simulink model "X1PFjicheng"  (R2024a)
settings: Solver=ode3  StartTime=0.0  StopTime=inf  FixedStep=0.05  RelTol=1e-3
undefined symbols (not defined in the file or in its folder): A0, Delta, down, Kdelta, P0, Td, Tj, ud, up, Waypoints, WPNum
libraries: slpidlib x2
(part 2 of 2)

== matlab function X1PFjicheng/AUV动力学模型1/MATLAB Function1 ==
  data: Xjiang input; Xshui input; Yshui input; Zshui input; Kshui input; Mshui input; Nshui input; Xduo input; Yduo input; Zduo input; Kduo input; Mduo input; Nduo input; Xjing input; Yjing input; dot_u output; dot_v output; dot_w output; dot_p output; Zjing input; Kjing input; Mjing input; u input; v input; w input; p input; q input; r input; dot_q output; dot_r output; mass input; Ix input; Iy input; Iz input; Xdot_u input; Ydot_v input; Ydot_p input; Ydot_r input; Zdot_w input; Zdot_q input; Kdot_p input; Kdot_v input; Kdot_r input; Mdot_q input; Mdot_w input; Ndot_v input; Ndot_p input; Ndot_r input
function [dot_u,dot_v,dot_w,dot_p,dot_q,dot_r]= fcn(Xjiang,Xshui,Yshui,Zshui,Kshui,Mshui,Nshui,Xduo,Yduo,Zduo,Kduo,Mduo,Nduo,Xjing,Yjing,Zjing,Kjing,Mjing,u,v,w,p,q,r,mass,Ix,Iy,Iz,Xdot_u,Ydot_v,Ydot_p,Ydot_r,Zdot_w,Zdot_q, ...
    Kdot_p,Kdot_v,Kdot_r,Mdot_q,Mdot_w,Ndot_v,Ndot_p,Ndot_r)

    
    dot_u=-(Xduo + Xjing + Xshui+Xjiang - mass*q*w + mass*r*v)/(Xdot_u - mass);

    dot_v= -(Ix*Iz*Yduo + Ix*Iz*Yjing + Ix*Iz*Yshui - Iz*Kdot_p*Yduo + Iz*Kduo*Ydot_p - Iz*Kdot_p*Yjing + Iz*Kjing*Ydot_p - Iz*Kdot_p*Yshui + Iz*Kshui*Ydot_p - ...
       Ix*Ndot_r*Yduo + Ix*Nduo*Ydot_r - Ix*Ndot_r*Yjing - Ix*Ndot_r*Yshui + Ix*Nshui*Ydot_r + Kdot_p*Ndot_r*Yduo - Kdot_p*Nduo*Ydot_r - Kdot_r*Ndot_p*Yduo + ...
       Kdot_r*Nduo*Ydot_p + Kduo*Ndot_p*Ydot_r - Kduo*Ndot_r*Ydot_p + Kdot_p*Ndot_r*Yjing - Kdot_r*Ndot_p*Yjing + Kjing*Ndot_p*Ydot_r - Kjing*Ndot_r*Ydot_p + ...
       Kdot_p*Ndot_r*Yshui - Kdot_p*Nshui*Ydot_r - Kdot_r*Ndot_p*Yshui + Kdot_r*Nshui*Ydot_p + Kshui*Ndot_p*Ydot_r - Kshui*Ndot_r*Ydot_p + Ix^2*Ydot_r*p*q - Iz^2*Ydot_p*q*r - ...
       Ix*Iy*Ydot_r*p*q - Ix*Kdot_p*Ydot_r*p*q + Ix*Kdot_r*Ydot_p*p*q + Iy*Kdot_p*Ydot_r*p*q - Iy*Kdot_r*Ydot_p*p*q + Iy*Iz*Ydot_p*q*r + Iy*Ndot_p*Ydot_r*q*r - Iy*Ndot_r*Ydot_p*q*r - ...
       Iz*Ndot_p*Ydot_r*q*r + Iz*Ndot_r*Ydot_p*q*r + Ix*Iz*mass*p*w - Ix*Iz*mass*r*u - Iz*Kdot_p*mass*p*w + Iz*Kdot_p*mass*r*u - Ix*Ndot_r*mass*p*w + Ix*Ndot_r*mass*r*u + ...
       Kdot_p*Ndot_r*mass*p*w - Kdot_p*Ndot_r*mass*r*u - Kdot_r*Ndot_p*mass*p*w + Kdot_r*Ndot_p*mass*r*u)/(Ix*Iz*Ydot_v - Iz*Kdot_p*Ydot_v + Iz*Kdot_v*Ydot_p - Ix*Ndot_r*Ydot_v + ...
       Ix*Ndot_v*Ydot_r + Kdot_p*Ndot_r*Ydot_v - Kdot_p*Ndot_v*Ydot_r - Kdot_r*Ndot_p*Ydot_v + Kdot_r*Ndot_v*Ydot_p + Kdot_v*Ndot_p*Ydot_r - Kdot_v*Ndot_r*Ydot_p - Ix*Iz*mass + Iz*Kdot_p*mass + ...
       Ix*Ndot_r*mass - Kdot_p*Ndot_r*mass + Kdot_r*Ndot_p*mass);

    dot_w= -(Iy*Zduo + Iy*Zjing + Iy*Zshui - Mdot_q*Zduo + Mduo*Zdot_q - Mdot_q*Zjing + Mjing*Zdot_q - Mdot_q*Zshui + Mshui*Zdot_q + Mdot_q*mass*p*v - Mdot_q*mass*q*u - Ix*Zdot_q*p*r + ...
       Iz*Zdot_q*p*r - Iy*mass*p*v + Iy*mass*q*u)/(Iy*Zdot_w - Mdot_q*Zdot_w + Mdot_w*Zdot_q - Iy*mass + Mdot_q*mass);
 
    dot_p=-(Iz*Kdot_v*Yduo - Iz*Kduo*Ydot_v + Iz*Kdot_v*Yjing - Iz*Kjing*Ydot_v + Iz*Kdot_v*Yshui - Iz*Kshui*Ydot_v + Kdot_r*Ndot_v*Yduo - Kdot_r*Nduo*Ydot_v - Kdot_v*Ndot_r*Yduo + ...
        Kdot_v*Nduo*Ydot_r + Kduo*Ndot_r*Ydot_v - Kduo*Ndot_v*Ydot_r + Kdot_r*Ndot_v*Yjing - Kdot_v*Ndot_r*Yjing + Kjing*Ndot_r*Ydot_v - Kjing*Ndot_v*Ydot_r + Kdot_r*Ndot_v*Yshui - ...
        Kdot_r*Nshui*Ydot_v - Kdot_v*Ndot_r*Yshui + Kdot_v*Nshui*Ydot_r + Kshui*Ndot_r*Ydot_v - Kshui*Ndot_v*Ydot_r + Iz*Kduo*mass + Iz*Kjing*mass + Iz*Kshui*mass + Kdot_r*Nduo*mass - ...
        Kduo*Ndot_r*mass - Kjing*Ndot_r*mass + Kdot_r*Nshui*mass - Kshui*Ndot_r*mass + Iz^2*Ydot_v*q*r - Iz^2*mass*q*r - Ix*Kdot_r*Ydot_v*p*q + Ix*Kdot_v*Ydot_r*p*q + Iy*Kdot_r*Ydot_v*p*q - ...
        Iy*Kdot_v*Ydot_r*p*q - Iy*Iz*Ydot_v*q*r + Iy*Ndot_r*Ydot_v*q*r - Iy*Ndot_v*Ydot_r*q*r - Iz*Ndot_r*Ydot_v*q*r + Iz*Ndot_v*Ydot_r*q*r + Ix*Kdot_r*mass*p*q - Iy*Kdot_r*mass*p*q + ...
        Iy*Iz*mass*q*r - Iy*Ndot_r*mass*q*r + Iz*Ndot_r*mass*q*r + Iz*Kdot_v*mass*p*w - Iz*Kdot_v*mass*r*u + Kdot_r*Ndot_v*mass*p*w - Kdot_r*Ndot_v*mass*r*u - Kdot_v*Ndot_r*mass*p*w + ...
        Kdot_v*Ndot_r*mass*r*u)/(Ix*Iz*Ydot_v - Iz*Kdot_p*Ydot_v + Iz*Kdot_v*Ydot_p - Ix*Ndot_r*Ydot_v + Ix*Ndot_v*Ydot_r + Kdot_p*Ndot_r*Ydot_v - Kdot_p*Ndot_v*Ydot_r - Kdot_r*Ndot_p*Ydot_v + ...
        Kdot_r*Ndot_v*Ydot_p + Kdot_v*Ndot_p*Ydot_r - Kdot_v*Ndot_r*Ydot_p - Ix*Iz*mass + Iz*Kdot_p*mass + Ix*Ndot_r*mass - Kdot_p*Ndot_r*mass + Kdot_r*Ndot_p*mass);
 
    dot_q=-(Mdot_w*Zduo - Mduo*Zdot_w + Mdot_w*Zjing - Mjing*Zdot_w + Mdot_w*Zshui - Mshui*Zdot_w + Mduo*mass + Mjing*mass + Mshui*mass - Mdot_w*mass*p*v + Mdot_w*mass*q*u + Ix*Zdot_w*p*r - ...
        Iz*Zdot_w*p*r - Ix*mass*p*r + Iz*mass*p*r)/(Iy*Zdot_w - Mdot_q*Zdot_w + Mdot_w*Zdot_q - Iy*mass + Mdot_q*mass);

   dot_r= -(Ix*Ndot_v*Yduo - Ix*Nduo*Ydot_v + Ix*Ndot_v*Yjing + Ix*Ndot_v*Yshui - Ix*Nshui*Ydot_v - Kdot_p*Ndot_v*Yduo + Kdot_p*Nduo*Ydot_v + Kdot_v*Ndot_p*Yduo - Kdot_v*Nduo*Ydot_p - ...
       Kduo*Ndot_p*Ydot_v + Kduo*Ndot_v*Ydot_p - Kdot_p*Ndot_v*Yjing + Kdot_v*Ndot_p*Yjing - Kjing*Ndot_p*Ydot_v + Kjing*Ndot_v*Ydot_p - Kdot_p*Ndot_v*Yshui + Kdot_p*Nshui*Ydot_v + Kdot_v*Ndot_p*Yshui - ...
       Kdot_v*Nshui*Ydot_p - Kshui*Ndot_p*Ydot_v + Kshui*Ndot_v*Ydot_p + Ix*Nduo*mass + Ix*Nshui*mass - Kdot_p*Nduo*mass + Kduo*Ndot_p*mass + Kjing*Ndot_p*mass - Kdot_p*Nshui*mass + Kshui*Ndot_p*mass - ...
       Ix^2*Ydot_v*p*q + Ix^2*mass*p*q + Ix*Iy*Ydot_v*p*q + Ix*Kdot_p*Ydot_v*p*q - Ix*Kdot_v*Ydot_p*p*q - Iy*Kdot_p*Ydot_v*p*q + Iy*Kdot_v*Ydot_p*p*q - Iy*Ndot_p*Ydot_v*q*r + Iy*Ndot_v*Ydot_p*q*r + Iz*Ndot_p*Ydot_v*q*r - ...
       Iz*Ndot_v*Ydot_p*q*r - Ix*Iy*mass*p*q - Ix*Kdot_p*mass*p*q + Iy*Kdot_p*mass*p*q + Iy*Ndot_p*mass*q*r - Iz*Ndot_p*mass*q*r + Ix*Ndot_v*mass*p*w - Ix*Ndot_v*mass*r*u - Kdot_p*Ndot_v*mass*p*w + Kdot_p*Ndot_v*mass*r*u + ...
       Kdot_v*Ndot_p*mass*p*w - Kdot_v*Ndot_p*mass*r*u)/(Ix*Iz*Ydot_v - Iz*Kdot_p*Ydot_v + Iz*Kdot_v*Ydot_p - Ix*Ndot_r*Ydot_v + Ix*Ndot_v*Ydot_r + Kdot_p*Ndot_r*Ydot_v - Kdot_p*Ndot_v*Ydot_r - Kdot_r*Ndot_p*Ydot_v + ...
       Kdot_r*Ndot_v*Ydot_p + Kdot_v*Ndot_p*Ydot_r - Kdot_v*Ndot_r*Ydot_p - Ix*Iz*mass + Iz*Kdot_p*mass + Ix*Ndot_r*mass - Kdot_p*Ndot_r*mass + Kdot_r*Ndot_p*mass);
 

	
end

== matlab function X1PFjicheng/AUV运动学模型1/MATLAB Function ==
  data: u input; ksi_dot output; v input; w input; phi input; theta input; psi input; eta_dot output; zeta_dot output
function [ksi_dot,eta_dot, zeta_dot] = fcn(u,v,w,phi,theta,psi)
ksi_dot=u*cos(psi)*cos(theta)+v*(cos(psi)*sin(theta)*sin(phi)-sin(psi)*cos(phi))+w*(sin(theta)*cos(psi)*sin(phi)+sin(psi)*sin(phi));
eta_dot=u*sin(psi)*cos(theta)+v*(sin(psi)*sin(theta)*sin(phi)+cos(phi)*cos(psi))+w*(sin(theta)*sin(psi)*cos(phi)-cos(psi)*sin(phi));
zeta_dot=-u*sin(theta)+v*cos(theta)*sin(phi)+w*cos(theta)*cos(phi);

end

== matlab function X1PFjicheng/Heading Autopilot/MATLAB Function3 ==
  data: in input; u output
function u = OrientationErrorDegSat(in)
if in > 180
    u = in - 360;
elseif in<-180
    u = in+360;
else
    u = in;
end

== matlab function X1PFjicheng/Compass/MATLAB Function ==
  data: in input; u output
function u = OrientationDegSat(in)
if in > 360
    u = in - 360;
elseif in<0
    u = in+360;
else
    u = in;
end

== matlab function X1PFjicheng/AUV动力学模型1/MATLAB Function2 ==
  data: p input; deg_p output; q input; r input; deg_q output; deg_r output
function [deg_p,deg_q,deg_r]= fcn(p,q,r)
deg_p=rad2deg(p);
deg_q=rad2deg(q);
deg_r=rad2deg(r);

== matlab function X1PFjicheng/卡舵设定/MATLAB Function ==
  data: u input; y output
function y = fcn(u)

y = deg2rad(u);

== matlab function X1PFjicheng/AUV动力学模型1/静力 ==
  data: P input; Xjing output; B input; theta input; Yjing output; Zjing output; Kjing output; Mjing output; phi input; Zg input; Zb input
 
function [Xjing,Yjing,Zjing,Kjing,Mjing]= fcn(P,B,theta,phi,Zg,Zb)

Xjing = -(P-B)*sin(theta);
Yjing = (P-B)*cos(theta)*sin(phi);
Zjing = (P-B)*cos(theta)*cos(phi);
Kjing = -(Zg*P-Zb*B)*cos(theta)*sin(phi);
Mjing =-(Zg*P-Zb*B)*sin(theta);

== matlab function X1PFjicheng/AUV动力学模型1/水动力1/MATLAB Function ==
  data: Xqq input; Xrr input; Xrp input; Xvr input; Xwq input; Xuu input; Xvv input; Xww input; Yp_p input; Ypq input; Yqr input; Yvq input; Ywp input; Ywr input; Yr input; Yp input; Yv_r input; Y0 input; Yv input; Yv_v input; Yvw input; Zpp input; Zrr input; Zrp input; Zvr input; Zvp input; Zq input; Zw_q input; Z0 input; Zw input; Zw_w input; Z_w input; Zww input; Kqr input; Kpq input; Kp_p input; Kp input; Kr input; Kvq input; Kwp input; Kwr input; K0 input; Kv input; Kv_v input; Kvw input; Mpp input; Mrr input; Mrp input; Mq_q input; Mvr input; Mvp input; Mq input; M_wq input; M0 input; Mw input; Mw_w input; M_w input; Mww input; Mvv input; Npq input; Nqr input; Nr_r input; Nwr input; Nwp input; Nvq input; Np input; Nr input; N_vr input; N0 input; Nv input; Nv_v input; Nvw input; u input; Xshui output; v input; w input; p input; q input; r input; Yshui output; Zshui output; Kshui output; Mshui output; Nshui output; rou input; L input
function [Xshui,Yshui,Zshui,Kshui,Mshui,Nshui]= fcn(Xqq,Xrr,Xrp,Xvr,Xwq,Xuu,Xvv,Xww, ...
    Yp_p ,Ypq,Yqr,Yvq,Ywp,Ywr,Yr,Yp,Yv_r ,Y0,Yv,Yv_v ,Yvw, ...
   Zpp,Zrr,Zrp,Zvr,Zvp,Zq,Zw_q,Z0,Zw,Zw_w,Z_w,Zww, ...
    Kqr,Kpq,Kp_p,Kp,Kr,Kvq,Kwp,Kwr,K0,Kv,Kv_v,Kvw, ...
  Mpp,Mrr,Mrp,Mq_q,Mvr,Mvp,Mq,M_wq,M0,Mw,Mw_w,M_w,Mww,Mvv, ...
    Npq,Nqr,Nr_r,Nwr,Nwp,Nvq,Np,Nr,N_vr,N0,Nv,Nv_v,Nvw, ...
    u,v,w,p,q,r,rou,L)
Xshui=0.5*rou*L^4*(Xqq*q ^2+Xrr*r^2+Xrp*r*p)+0.5*rou*L^3*(Xvr*v*r*+Xwq*w*q)+0.5*rou*L^2*(Xuu*u*u+Xvv*v*v+Xww*w*w);
Yshui=0.5*rou*L^4*(Yp_p*p*abs(p)+Ypq*p*q+Yqr*q*r)+0.5*rou*L^3*(Yvq*v*q+Ywp*w*p+Ywr*w*r)+0.5*rou*L^3*(Yr*u*r+Yp*u*p+Yv_r*sign(v)*abs(sqrt(v^2+w^2))*abs(r))+0.5*rou*L^2*(Y0*u*u+Yv*u*v+Yv_v*v*abs(sqrt(v^2+w^2))+Yvw*v*w);
Zshui=0.5*rou*L^4*(Zpp*p*p+Zrr*r*r+Zrp*r*p)+0.5*rou*L^3*(Zvr*v*r+Zvp*v*p)+0.5*rou*L^3*(Zq*u*q+Zw_q*sign(w)*abs(sqrt(v^2+w^2))*abs(q))+0.5*rou*L^2*(Z0*u*u+Zw*u*w+Zw_w*w*abs(sqrt(v^2+w^2)) +Z_w*u*abs(w)+Zww*abs(w*sqrt(v^2+w^2)));
Kshui=0.5*rou*L^5*(Kqr*q*r+Kpq*p*q+Kp_p*p*abs(p))+0.5*rou*L^4*(Kp*u*p+Kr*u*r+Kvq*v*q+Kwp*w*p+Kwr*w*r)+0.5*rou*L^3*(K0*u*u+Kv*u*v+Kv_v*v*abs(sqrt(v^2+w^2))+Kvw*v*w);
Mshui=0.5*rou*L^5*(Mpp*p*p+Mrr*r*r+Mrp*r*p+Mq_q*q*abs(q))+0.5*rou*L^4*(Mvr*v*r+Mvp*v*p+Mq*u*q+M_wq*abs(sqrt(v^2+w^2))*q)+0.5*rou*L^3*(M0*u*u+Mw*u*w+Mw_w*w*abs(sqrt(v^2+w^2))+M_w*u*abs(w)+Mww*abs(w*sqrt(v^2+w^2))+Mvv*v*v);
Nshui=0.5*rou*L^5*(Npq*p*q+Nqr*q*r+Nr_r*r*abs(r))+0.5*rou*L^4*(Nwr*w*r+Nwp*w*p+Nvq*v*q+Np*u*p+Nr*u*r+N_vr*abs(sqrt(v^2+w^2))*r)+0.5*rou*L^3*(N0*u*u+Nv*u*v+Nv_v*v*abs(sqrt(v^2+w^2))+Nvw*v*w);

== matlab function X1PFjicheng/卡舵设定/MATLAB Function4 ==
  data: u input; y output
function y = fcn(u)

y = deg2rad(u);

== matlab function X1PFjicheng/Coupled3DLOS/CoupledLOS ==
  data: ye input; ze input; R_FN input; delta_max input; delta_min input; nanmda input; Gamma_d output; Chi_d output; min input; max input; Delta output
function [Gamma_d,Chi_d,Delta] = fcn(ye,ze,R_FN,delta_max,delta_min,nanmda,min,max)

if ye>min && ye<max
Delta=(delta_max-delta_min)*exp(-nanmda*ye^2)+delta_min;
elseif ye<=min 
    Delta=delta_min;
else 
    Delta=delta_max;
end

LOS_F = [Delta;ye;ze];
LOS_N = R_FN*LOS_F;
Gamma_d = atan2(LOS_N(2),LOS_N(1));
%Gamma_d = atan2(LOS_N(2),sign(LOS_N(1))*sqrt(LOS_N(1)*LOS_N(1)+LOS_N(3)*LOS_N(3)));
if Gamma_d<0
    Gamma_d = Gamma_d+2*pi;
end
Gamma_d = Gamma_d*180/pi;
Chi_d = -atan(LOS_N(3)/sqrt(LOS_N(1)^2+LOS_N(2)^2))*180/pi;
%Chi_d = -atan(LOS_N(3)/abs(LOS_N(1)))*180/pi;
end

== matlab function X1PFjicheng/Track Error Cal ==
  data: ye output; ze output; P input; WP input; Gamma_p input; Chi_p input; R_FN output; xe output
function [ye,ze,R_FN,xe] = fcn(P,WP,Gamma_p,Chi_p)
sg = sin(Gamma_p);cg = cos(Gamma_p);
sc = sin(Chi_p);cc = cos(Chi_p);
R_FN = [cg*cc -sg cg*sc; sg*cc cg sg*sc; -sc 0 cc];
R_NF = R_FN';
E_F = R_NF*(WP-P);

xe = E_F(1);
ye = E_F(2);
ze = E_F(3);
end

== matlab function X1PFjicheng/AUV动力学模型1/舵力 ==
  data: u input; Xduo output; Yduo output; Zduo output; Kduo output; Mduo output; Nduo output; delta1 input; delta2 input; delta3 input; delta4 input; X_delta input; Y_delta input; Z_delta input; K_delta input; M_delta input; N_delta input
function [Xduo, Yduo, Zduo, Kduo, Mduo, Nduo] = fcn(u, delta1, delta2, delta3, delta4, X_delta, Y_delta, Z_delta, K_delta, M_delta, N_delta)
if delta1==delta2 && delta2==delta3  && delta3==delta4 && delta4==90*pi/180
    Xduo=-(1141*u^2+118.2*u-6.442);
    Yduo=0;
    Zduo=0;
    Kduo=0;
    Mduo=0;
    Nduo=0;
else
Xduo= X_delta*u^2*(delta1^2+delta2^2+delta3^2+delta4^2);
Yduo=Y_delta*u^2*(delta1+delta2)-Y_delta*u^2*(delta3+delta4);
Zduo=Z_delta*u^2*(delta1+delta2+delta3+delta4);
Kduo=K_delta*u^2*(delta1+delta3)-K_delta*u^2*(delta2+delta4);
Mduo=M_delta*u^2*(delta1+delta2+delta3+delta4);
Nduo=N_delta*u^2*(delta1+delta2)-N_delta*u^2*(delta3+delta4);
end

== matlab function X1PFjicheng/Waypoint Switch/If Action Subsystem1/MATLAB Function1 ==
  data: WP output; WPSEQ input; WPID input; Gamma_p output; Chi_p output; P0 input; error output
function [WP,Gamma_p,Chi_p,error] = fcn(WPSEQ,WPID,P0)
WP = WPSEQ(WPID,:)';

if WPID == 1
    dx = WPSEQ(1,1)-P0(1);dy = WPSEQ(1,2)-P0(2);dz = WPSEQ(1,3)-P0(3);
else
    dp = WPSEQ(WPID,:)-WPSEQ(WPID-1,:);
    dx = dp(1);dy = dp(2);dz = dp(3);
end

Gamma_p = atan2(dy,dx);
Chi_p = -atan(dz/sqrt(dx*dx+dy*dy));

if Gamma_p<0
    Gamma_p = Gamma_p + 2*pi;
end
  
    % 获取上一个航点坐标
   
    if WPID==1
    x = WP(1) - P0(1);
    y = WP(2) - P0(2);
    z = WP(3) - P0(3);
      error = sqrt(x^2 + y^2 + z^2);
    else
         prevWP = WPSEQ(WPID - 1, :); % 上一个航点 [x1, y1, z1]
    % 计算相邻两个航点之间的欧几里得距离（位置误差）
    x = WP(1) - prevWP(1);
    y = WP(2) - prevWP(2);
    z = WP(3) - prevWP(3);
    
    % 位置误差
    error = sqrt(x^2 + y^2 + z^2);
    end

== matlab function X1PFjicheng/Heading Autopilot/MATLAB Function ==
  data: e input; akp output; u input; kp input
function akp = fcn(e,u,kp)
if u==0
akp = e*kp/((u+0.01));
else 
   akp = e*kp/(u);
end

== matlab function X1PFjicheng/Heading Autopilot/MATLAB Function1 ==
  data: e input; akd output; u input; kd input
function akd = fcn(e,u,kd)
if u==0
akd = e*kd/(u+0.01);
else 
   akd = e*kd/u;
end

== matlab function X1PFjicheng/Heading Autopilot/MATLAB Function2 ==
  data: e input; akp output; u input; kp input
function akp = fcn(e,u,kp)
if u==0
akp = e*kp/((u+0.01));
else 
   akp = e*kp/(u);
end

== matlab function X1PFjicheng/Pitch Autopilot/MATLAB Function ==
  data: e input; u input; akp output; kp input
function akp = fcn(e,u,kp)
if u==0
akp = e*kp;
else 
   akp = e*kp/(u);
end

== matlab function X1PFjicheng/Pitch Autopilot/MATLAB Function1 ==
  data: e input; u input; akd output; kd input
function akd = fcn(e,u,kd)
if u==0
akd = e*kd;
else 
   akd = e*kd/(u);
end

== matlab function X1PFjicheng/卡舵设定/MATLAB Function5 ==
  data: delta_in input; delta_out output; t input; tk input; delta_k input
function delta_out = fcn(delta_in,t,tk,delta_k)
%t:clock
%tk:卡舵时间t
%delta_k:卡舵舵角
if t<tk
    delta_out=delta_in;
else
    delta_out=delta_k;
end

== matlab function X1PFjicheng/卡舵设定/MATLAB Function6 ==
  data: u input; y output
function y = fcn(u)

y = deg2rad(u);

== matlab function X1PFjicheng/MATLAB Function1 ==
  data: ud input; R input; Rd input; Rm input; k input; u output; delta_d input
function u = fcn(ud,R,Rd,Rm,k,delta_d)
if abs(delta_d)>=Rd && abs(delta_d)<=Rm
    u=ud;
% elseif abs(delta_d)>=R && abs(delta_d)<Rd
%     u=((1-k)/(Rd-R)*(delta_d-Rd)+1)*ud;
elseif abs(delta_d)>Rm
 u=k*ud;
else
    u=k*ud;
end

== matlab function X1PFjicheng/MATLAB Function3 ==
  data: u input; Xjiang output; n input; uliu input
function Xjiang = fcn(u,n,uliu)
Xjiang=-41.48*(u+uliu)^2-207.7*n*(u+uliu)/60+450.4*n^2/3600;

== matlab function X1PFjicheng/Pitch Autopilot1/MATLAB Function ==
  data: e input; akp output; u input; kp input
function akp = fcn(e,u,kp)

akp = e*(kp-0.3*u);

== matlab function X1PFjicheng/Pitch Autopilot1/MATLAB Function1 ==
  data: e input; akd output; u input; kd input
function akd = fcn(e, u, kd)
akd=e*(0.8*u+kd);

== matlab function X1PFjicheng/Pitch Autopilot1/MATLAB Function2 ==
  data: e input; akd output; u input; ki input
function akd = fcn(e,u,ki)

akd = e*(u+1.5)/ki;

== matlab function X1PFjicheng/卡舵判定 ==
  data: delta_exp1 input; delta output; delta_in1 input; delta_exp2 input; delta_in2 input; delta_exp3 input; delta_in3 input; delta_exp4 input; delta_in4 input; M input; N input; M_delta input; N_delta input; u input; P output
function [delta,P] = fcn(delta_exp1,delta_in1,delta_exp2,delta_in2,delta_exp3,delta_in3,delta_exp4,delta_in4,M,N,M_delta,N_delta,u)
%B:舵角矩阵   tau:期望力矩    delta：四个舵角
tau=[M;N];
delta=[0;0;0;0];

%四个舵正常工作 
if delta_exp1==delta_in1 && delta_exp2==delta_in2 && delta_exp3==delta_in3 && delta_exp4==delta_in4 
B =[
    M_delta,M_delta,M_delta,M_delta;
    N_delta, N_delta, -N_delta, -N_delta]*u^2 ;
    delta=B'*inv(B*B')*tau;
    P=39647.00;

  %舵1卡舵角
  elseif delta_exp1~=delta_in1 && delta_exp2==delta_in2 && delta_exp3==delta_in3 && delta_exp4==delta_in4 
    B =[
    M_delta,M_delta,M_delta;
    N_delta, -N_delta, -N_delta]*u^2 ;
    deltanew=B'*inv(B*B')*[M-M_delta*delta_in1*u*u;N-N_delta*delta_in1*u*u];%减去卡舵舵角提供的力矩，1、3、4舵重新分配
    delta=[delta_in1;deltanew(1,:);deltanew(2,:);deltanew(3,:)];
    P=39647.00;
  %舵2卡舵角
elseif delta_exp1==delta_in1 && delta_exp2~=delta_in2 && delta_exp3==delta_in3 && delta_exp4==delta_in4 
    B =[ 
    M_delta,M_delta,M_delta;
    N_delta, -N_delta, -N_delta]*u^2 ;
    deltanew=B'*inv(B*B')*[M-M_delta*delta_in2*u*u;N-N_delta*delta_in2*u*u];%减去卡舵舵角提供的力矩，1、3、4舵重新分配
    delta=[deltanew(1,:);delta_in2;deltanew(2,:);deltanew(3,:)];
    P=39647.00;
  %舵3卡舵角
elseif delta_exp1==delta_in1 && delta_exp2==delta_in2 && delta_exp3~=delta_in3 && delta_exp4==delta_in4 
   B =[
    M_delta,M_delta,M_delta;
    N_delta, N_delta,-N_delta]*u^2 ;
    deltanew=B'*inv(B*B')*[M-M_delta*delta_in3*u*u;N+N_delta*delta_in3*u*u];%减去卡舵舵角提供的力矩，1、2、4舵重新分配
    delta=[deltanew(1,:);deltanew(2,:);delta_in3;deltanew(3,:)]; 
    P=39647.00;
%舵4卡舵角
elseif delta_exp1==delta_in1 && delta_exp2==delta_in2 && delta_exp3==delta_in3 && delta_exp4~=delta_in4 
B =[
    M_delta,M_delta,M_delta;
    N_delta, N_delta, -N_delta]*u^2 ;   
    deltanew=B'*inv(B*B')*[M-M_delta*delta_in4*u*u;N+N_delta*delta_in4*u*u];%减去卡舵舵角提供的力矩，1、2、3舵重新分配
    delta=[deltanew(1,:);deltanew(2,:);deltanew(3,:);delta_in4];  
    P=39647.00;
   %卡双舵
   %舵1、4卡舵角
elseif delta_exp1~=delta_in1 && delta_exp2==delta_in2 && delta_exp3==delta_in3 && delta_exp4~=delta_in4 
B =[
   M_delta,M_delta;
    N_delta, -N_delta]*u^2 ;   
    deltanew=B'*inv(B*B')*[M-(M_delta*(delta_in1+delta_in4)*u*u);N-(N_delta*(delta_in1-delta_in4)*u*u)];%减去卡舵舵角提供的力矩，2、3舵重新分配
    delta=[delta_in1;deltanew(1,:);deltanew(2,:);delta_in4];
    P=39647.00;
 %舵1、3卡舵角
 elseif delta_exp1~=delta_in1 && delta_exp2==delta_in2 && delta_exp3~=delta_in3 && delta_exp4==delta_in4 
 B =[
    M_delta,M_delta;
    N_delta, -N_delta]*u^2 ;   
    deltanew=B'*inv(B*B')*[M-(M_delta*(delta_in3+delta_in1)*u*u);N-(N_delta*(delta_in1-delta_in3)*u*u)];%减去卡舵舵角提供的力矩，1、2、3舵重新分配
    delta=[delta_in1;deltanew(1,:);delta_in3;deltanew(2,:);]; 
    P=39647.00;
%舵2、3卡舵角
elseif delta_exp1==delta_in1 && delta_exp2~=delta_in2 && delta_exp3~=delta_in3 && delta_exp4==delta_in4 
 B =[
    M_delta,M_delta;
    N_delta, -N_delta]*u^2 ;   
    deltanew=B'*inv(B*B')*[M-(M_delta*(delta_in3+delta_in2)*u*u);N-(N_delta*(delta_in2-delta_in3)*u*u)];%减去卡舵舵角提供的力矩，1、2、3舵重新分配
    delta=[deltanew(1,:);delta_in2;delta_in3;deltanew(2,:)]; 
    P=39647.00;
 %舵2、4卡舵角
elseif delta_exp1==delta_in1 && delta_exp2~=delta_in2 && delta_exp3==delta_in3 && delta_exp4~=delta_in4 
 B =[
    M_delta,M_delta;
    N_delta, -N_delta]*u^2 ;   
    deltanew=B'*inv(B*B')*[M-(M_delta*(delta_in4+delta_in2)*u*u);N-(N_delta*(delta_in2-delta_in4)*u*u)];%减去卡舵舵角提供的力矩，1、2、3舵重新分配
    delta=[deltanew(1,:);delta_in2;deltanew(2,:);delta_in4]; 
%卡对角舵
P=39647.00;
%卡1、2
elseif delta_exp1~=delta_in1 && delta_exp2~=delta_in2 && delta_exp3==delta_in3 && delta_exp4==delta_in4 
   
     P=39647.00-200;
elseif delta_exp1==delta_in1 && delta_exp2==delta_in2 && delta_exp3~=delta_in3 && delta_exp4~=delta_in4 
  
     P=39647.00-200;
else
  
    P=39647.00-200;

end

== matlab function X1PFjicheng/卡舵设定/MATLAB Function1 ==
  data: delta_in input; delta_out output; t input; tk input; delta_k input
function delta_out = fcn(delta_in,t,tk,delta_k)
%t:clock
%tk:卡舵时间t
%delta_k:卡舵舵角
if t<tk
    delta_out=delta_in;
else
    delta_out=delta_k;
end

== matlab function X1PFjicheng/卡舵设定/MATLAB Function2 ==
  data: u input; y output
function y = fcn(u)

y = deg2rad(u);

== matlab function X1PFjicheng/卡舵设定/MATLAB Function3 ==
  data: delta_in input; delta_out output; t input; tk input; delta_k input
function delta_out = fcn(delta_in,t,tk,delta_k)
%t:clock
%tk:卡舵时间t
%delta_k:卡舵舵角
if t<tk
    delta_out=delta_in;
else
    delta_out=delta_k;
end

== matlab function X1PFjicheng/卡舵设定/MATLAB Function7 ==
  data: delta_in input; delta_out output; t input; tk input; delta_k input
function delta_out = fcn(delta_in,t,tk,delta_k)
%t:clock
%tk:卡舵时间t
%delta_k:卡舵舵角
if t<tk
    delta_out=delta_in;
else
    delta_out=delta_k;
end

== matlab function X1PFjicheng/AUV动力学模型1/MATLAB Function3 ==
  data: rou input; rou_out output; t input; t_d input; rou_d input
function rou_out = fcn(rou,t,t_d,rou_d)

if t<t_d
    rou_out=rou;
else
    rou_out=rou_d;
end

== matlab function X1PFjicheng/AUV动力学模型1/判定是否抛载 ==
  data: Z input; y output; waypoints input; P input; pao input; y input; delta_z input
function y = fcn(Z, waypoints, P, pao,y,delta_z)
    % 输入说明：
    % Z - 当前状态值
    % waypoints - 包含参考值的向量
    % P - 原始重量
    % pao - 抛载重量
    % y - 当前重量
    
   

    % 判断是否需要抛载
    if Z - waypoints(3) >= delta_z && y==P
        y = P - pao;
    elseif Z - waypoints(3)<=delta_z && y==P-pao
        y=P-pao; 
    elseif Z - waypoints(3) <delta_z-4.8 && y~=P
        y = P;
    end
end

== matlab function X1PFjicheng/MATLAB Function4 ==
  data: ud input; T input; Tj input; t input; ue output; Td input

% function ue = fcn(ud, ur, T, Tj)
% 
%     if T >= Tj && ur <= 0
%         ue = ud; % 情况 2: T >= Tj 且 ur == 0
%     elseif T>=Tj && ur>0
%         ue=0;
%     else
%         ue = ud; % 情况 3: 其他情况（包括 T < Tj）
%     end
% end

function ue = fcn(ud, T, Tj,t,Td)

if   T>Td
    ue=0.01;
elseif T<Tj
    ue=ud;
elseif T>=Tj && T<=Tj+t
    ue=0;

else
    ue=ud;
end

== matlab function X1PFjicheng/MATLAB Function5 ==
  data: ue input; d1 input; d2 input; d3 input; d4 input; delta1 output; P input; delta2 output; delta3 output; delta4 output
function [delta1,delta2,delta3,delta4] = fcn(ue,d1,d2,d3,d4,P)

%%
if P<39647.00*9.8
%   d=[d1 d2 d3 d4];
%  delta = zeros(1,4);
% % 根据A中的元素设置delta值
% for i = 1:length(A)
%     if isinf(A(i))
%         delta(i) =-10*pi/180;  % 如果A(i)是inf，delta(i)等于A(i)
%     else
%         delta(i) =d(i);  % 如果A(i)是数字，delta(i)等于10
%     end
% end
%     delta1=delta(1);
%     delta2=delta(2);
%     delta3=delta(3);
%     delta4=delta(4);
% 
     delta1=-20*pi/180;
     delta2=-20*pi/180;
     delta3=-20*pi/180;
     delta4=-20*pi/180;

elseif ue==0
    delta1=90*pi/180;
    delta2=90*pi/180;
    delta3=90*pi/180;
    delta4=90*pi/180;
else
    delta1=d1;
    delta2=d2;
    delta3=d3;
    delta4=d4;
end

== matlab function X1PFjicheng/转向航速系数 ==
  data: u input; k output
function k = fcn(u)
if u<=2.5
    k=1;
else
    k=1.2/u;

end

== matlab function X1PFjicheng/MATLAB Function6 ==
  data: T input; Kdelta input; status output; Td input; Tj input; X input; Y input; Waypoints input; P input; down input; up input
function status = fcn(T,Kdelta,Td,Tj,X,Y,Waypoints,P,down,up)
%0:正常
%1：急停
%2：上浮
%3：下潜
%4：避障
%5：卡舵
%6：掉深
%7：抛载
Tk=min(Kdelta);
t1=min(Tk,Tj);
t2=max(Tk,Tj);
if  P<39647.00*9.8 %抛载
    status=7;
elseif T>=t1 && T<t2%卡舵
    if t1==Tk
     status=5;
    else
        status=1;
    end
elseif T>=t2%急停
    if t2==Tj
    status=1;
    else
        status=5;
    end
elseif T>Td && P==39647.00*9.8%掉深
    status=6;
elseif X<=Waypoints(down-1,1)+10 && X>=Waypoints(down+1,1)-10 && Y>=min(Waypoints(down-1,2),Waypoints(down+1,2)) && Y<max(Waypoints(down-1,2),Waypoints(down+1,2))%下潜
    status=3;
elseif X<=Waypoints(up-1,1)+10 && X>=Waypoints(up+1,1)-10 && Y>=min(Waypoints(up-1,2),Waypoints(up+1,2)) && Y<max(Waypoints(up-1,2),Waypoints(up+1,2)) %上浮
    status=2;
elseif X>=470-3 && X<=560+10 && Y>=90 && Y<1820   %避障
    status=4;

else
    status=0; %正常运行
end

== matlab function X1PFjicheng/Coupled3DLOS/MATLAB Function ==
  data: u input; delta output
function delta = fcn(u)
if u<=3.5 && u~=3
    delta=0.6477*sin(u-pi)-0.2364*(u-10)^2+79.6038;
elseif u==3
    delta=36;
elseif u>3.5 && u<=5.3
    delta=35;
elseif u>5.3 && u<=6.5
    delta=40;
elseif u>6.5 && u<=7.5
   delta=50;
else
    delta=160;
end

== matlab function X1PFjicheng/Pitch Autopilot/MATLAB Function2 ==
  data: e input; u input; akp output; ki input
function akp = fcn(e,u,ki)
if u==0
akp = e*ki;
else 
   akp = e*ki/(u);
end

== matlab function X1PFjicheng/AUV动力学模型1/MATLAB Function4 ==
  data: P input; y output; P1 input
function y = fcn(P,P1)

y = min(P1,P);
